simulink model "inv_dyn_scheme"  (R2020a)
settings: Solver=VariableStepAuto  StartTime=0.0  StopTime=10  RelTol=1e-3
values from neighbouring files (symbols this model uses):
  q0 = [0 0 0 0 0 0 ]    [JoinScript.m]    (also in alldata.mat = [0 0 0 0 0 0]; model_script.m = q; script_trj_q.m = [0 0 0 0 0 0]*pi/180)
settings Model: Creator=Administrator  LastModifiedBy=doble
settings DataIOCC: SaveFormat=Array  SaveOutput=off  SignalLogging=off  DSMLogging=off  SaveTime=off  ReturnWorkspaceOutputs=off

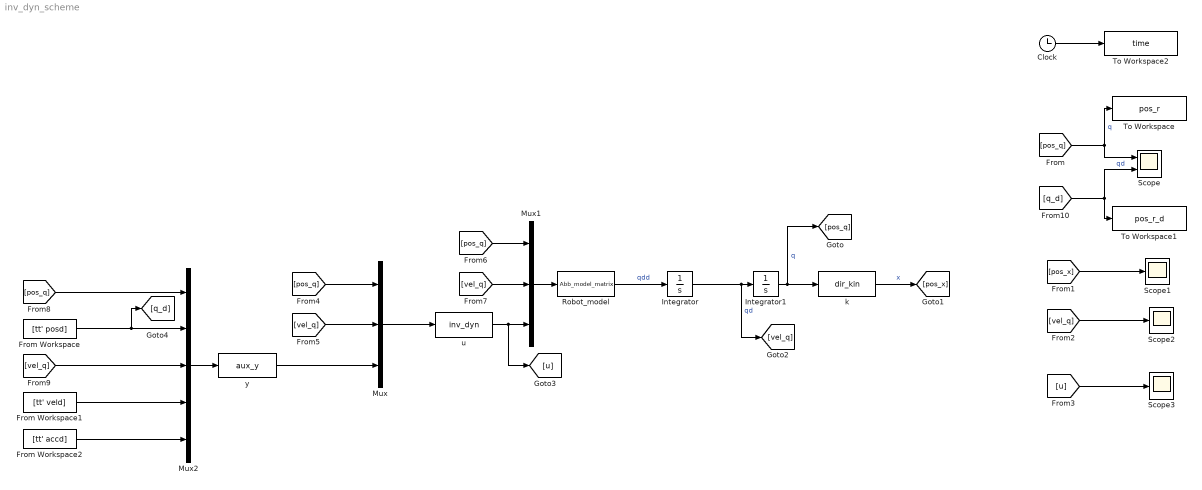
== system inv_dyn_scheme ==
  Clock : Clock
  From Workspace : FromWorkspace  VariableName=[tt' posd]
  From Workspace1 : FromWorkspace  VariableName=[tt' veld]
  From Workspace2 : FromWorkspace  VariableName=[tt' accd]
  Integrator : Integrator
  Integrator1 : Integrator  InitialCondition=q0
  Mux : Mux  Inputs=[6 6 6]
  Mux1 : Mux  Inputs=[6 6 6]
  Mux2 : Mux  Inputs=[6 6 6 6 6]
  Robot_model : MATLABFcn  MATLABFcn=Abb_model_matrix  OutputDimensions=6
  Scope : Scope  NumInputPorts=2
  Scope1 : Scope
  Scope2 : Scope
  Scope3 : Scope
  To Workspace : ToWorkspace  VariableName=pos_r  SampleTime=-1
  To Workspace1 : ToWorkspace  VariableName=pos_r_d  SampleTime=-1
  To Workspace2 : ToWorkspace  VariableName=time  SampleTime=-1
  k : MATLABFcn  MATLABFcn=dir_kin
  u : MATLABFcn  MATLABFcn=inv_dyn  OutputDimensions=6
  y : MATLABFcn  MATLABFcn=aux_y
  wires:
  Robot_model/1 -> Integrator/1  "qdd"
  Integrator/1 -> [vel_q], Integrator1/1  "qd"
  Integrator1/1 -> [pos_q], k/1  "q"
  k/1 -> [pos_x]  "x"
  Mux/1 -> u/1
  u/1 -> Mux1/3, [u]
  [pos_q] -> Mux/1
  [vel_q] -> Mux/2
  Mux1/1 -> Robot_model/1
  [pos_q] -> Mux1/1
  [vel_q] -> Mux1/2
  y/1 -> Mux/3
  Mux2/1 -> y/1
  [pos_q] -> Mux2/1
  From Workspace/1 -> [q_d], Mux2/2
  [vel_q] -> Mux2/3
  From Workspace1/1 -> Mux2/4
  From Workspace2/1 -> Mux2/5
  [pos_q] -> Scope/1, To Workspace/1  "q"
  [q_d] -> To Workspace1/1, Scope/2  "qd"
  Clock/1 -> To Workspace2/1
  [pos_x] -> Scope1/1
  [vel_q] -> Scope2/1
  [u] -> Scope3/1
